simulink model "DCMACHINE"  (R2024b)
settings: Solver=VariableStepAuto  StartTime=0.0  StopTime=3  RelTol=1e-3
libraries: spsDCVoltageSourceLib x2, spsVoltageMeasurementLib x2, spsDCMachineLib x1, sps_lib x1
settings Model: Creator=495ka  LastModifiedBy=495ka
settings SolverCC: ZeroCrossAlgorithm=Adaptive
settings DebuggingCC: IgnoredZcDiagnostic=none

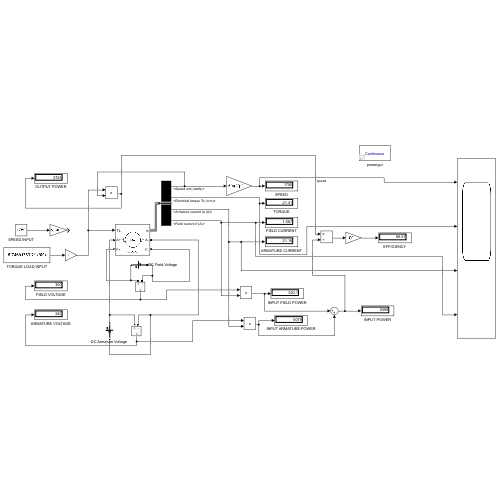
[thumbnail: Simulink's stored preview of the top-level diagram]
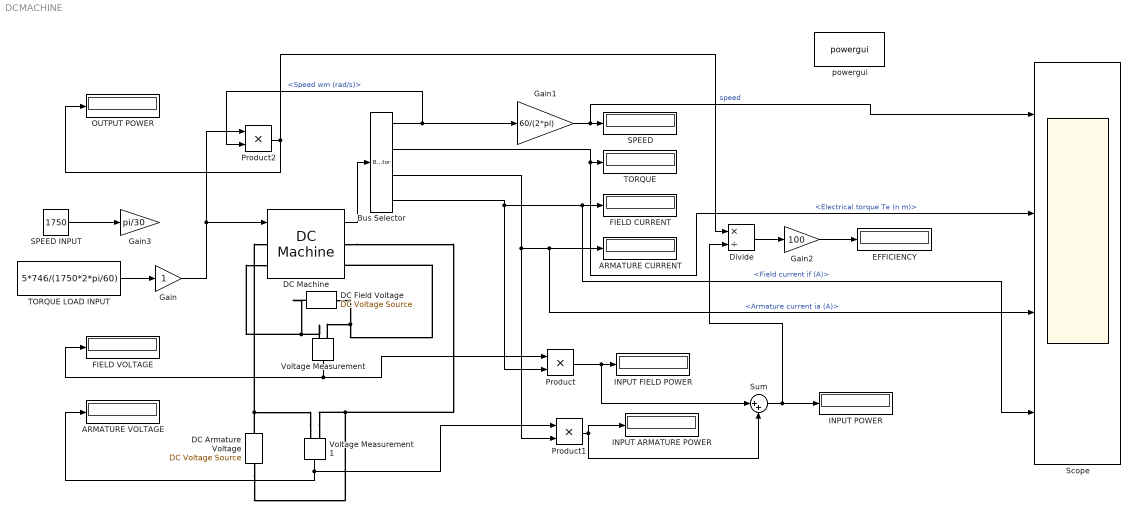
== system DCMACHINE ==
  ARMATURE CURRENT : Display
  ARMATURE VOLTAGE : Display
  Bus Selector : BusSelector  OutputSignals=Speed wm (rad/s),Electrical torque Te (n m),Armature current ia (A),Field current if (A)
  "DC Armature Voltage " : spsDCVoltageSourceLib/DC Voltage Source  Amplitude=240  Measurements=None
  DC Field Voltage : spsDCVoltageSourceLib/DC Voltage Source  Amplitude=300  Measurements=None
  DC Machine : spsDCMachineLib/DC Machine  PresetModel=01: 5HP 240V 1750RPM Field:300V  MechanicalLoad=Torque TL  FieldType=Wound  ShowDetailedParameters=on  MeasurementBus=off  RLa=[2.581 0.028]  RLf=[281.2 156]  Laf=0.9483  MachineConstant=Torque constant (N.m/A)  Ke=1.8  Kt=1.8  J=0.02215  Bm=0.002953  Tf=0.5161  w0=1  Ifinit=1.06685633001422  TsPowergui=0  TsBlock=-1
  Divide : Product  Inputs=*/
  EFFICIENCY : Display
  FIELD CURRENT : Display
  FIELD VOLTAGE : Display
  Gain : Gain
  Gain1 : Gain  Gain=60/(2*pi)
  Gain2 : Gain  Gain=100
  Gain3 : Gain  Gain=pi/30
  INPUT ARMATURE POWER : Display
  INPUT FIELD POWER : Display
  INPUT POWER : Display
  OUTPUT POWER : Display
  Product : Product
  Product1 : Product
  Product2 : Product
  SPEED : Display
  SPEED INPUT : Constant  Value=1750
  Scope : Scope  NumInputPorts=4
  Sum : Sum  Inputs=|++
  TORQUE : Display
  TORQUE LOAD INPUT : Constant  Value=5*746/(1750*2*pi/60)
  Voltage Measurement : spsVoltageMeasurementLib/Voltage Measurement  PhasorSimulation=off  OutputType=Complex  PSBequivalent=0
  Voltage Measurement1 : spsVoltageMeasurementLib/Voltage Measurement  PhasorSimulation=off  OutputType=Complex  PSBequivalent=0
  powergui : sps_lib/powergui  Priority=1  SimulationMode=Continuous  SampleTime=50e-6  frequency=60  Iterations=50  frequencyindice=0  Pbase=100e6  ErrMax=1e-4  UnitsV=kV  UnitsW=MW  buscounter=0  FunctionMessages=off  echomessages=off  EnableUseOfTLC=off  CurrentSourceSwitches=off  DisableSnubberDevices=off  DisableRonSwitches=off  DisableVfSwitches=off  DisplayEquations=off  AutomaticDiscreteSolvers=off  SolverType=Tustin/Backward Euler (TBE)  Interpol=off  ExternalGateDelay=off  methode=off  Ts=100  x0status=blocks  SPID=on  SwTol=0  HookPort=off  NonlinearTolerance=1e-4  nMaxIteration=100  ContinueOnMaxIteration=off  RestoreLinks=warning  ResistiveCurrentMeasurement=off  Frange=[0:2:500]  Ylog=off  Xlog=on  ShowGrid=off  save=off  variable=ZData  structure=0  ZoomFFT=off  StartTime=0.0  cycles=1  DisplayStyle=1  fundamental=60  FreqAxis=off  MaxFrequency=1000  frequencyindicesteady=1  RmsSteady=1  display=off
  wires:
  DC Machine/1 -> Bus Selector/1
  Bus Selector/1 -> Gain1/1, Product2/2  "<Speed wm (rad/s)>"
  Bus Selector/2 -> TORQUE/1, Scope/2  "<Electrical torque Te (n m)>"
  Bus Selector/4 -> Product/2, Scope/4, FIELD CURRENT/1  "<Field current if (A)>"
  Bus Selector/3 -> Product1/2, Scope/3, ARMATURE CURRENT/1  "<Armature current ia (A)>"
  Gain1/1 -> Scope/1, SPEED/1  "speed"
  Voltage Measurement/1 -> FIELD VOLTAGE/1, Product/1
  Voltage Measurement1/1 -> Product1/1, ARMATURE VOLTAGE/1
  Product/1 -> Sum/1, INPUT FIELD POWER/1
  Product1/1 -> INPUT ARMATURE POWER/1, Sum/2
  Sum/1 -> Divide/2, INPUT POWER/1
  Product2/1 -> Divide/1, OUTPUT POWER/1
  Divide/1 -> Gain2/1
  Gain2/1 -> EFFICIENCY/1
  SPEED INPUT/1 -> Gain3/1
  TORQUE LOAD INPUT/1 -> Gain/1
  Gain/1 -> DC Machine/1, Product2/1
  connections:
  Voltage Measurement/LConn1 -- DC Field Voltage/RConn1 -- DC Machine/LConn2
  Voltage Measurement1/LConn2 -- DC Machine/RConn1 -- "DC Armature Voltage "/LConn1
  Voltage Measurement/LConn2 -- DC Machine/RConn2 -- DC Field Voltage/LConn1
  Voltage Measurement1/LConn1 -- "DC Armature Voltage "/RConn1 -- DC Machine/LConn1
